simulink model "filling_model"  (R2020b)
settings: Solver=FixedStepAuto  StartTime=tank_pressure.time(1)  StopTime=tank_pressure.time(end)  FixedStep=1  RelTol=1e-3
undefined symbols (not defined in the file or in its folder): bar_to_Pa, eta_Faraday_builtin, F, k, ncell, R, tank_pressure, Ttank, Vtank
settings Model: Creator=keske  LastModifiedBy=keske

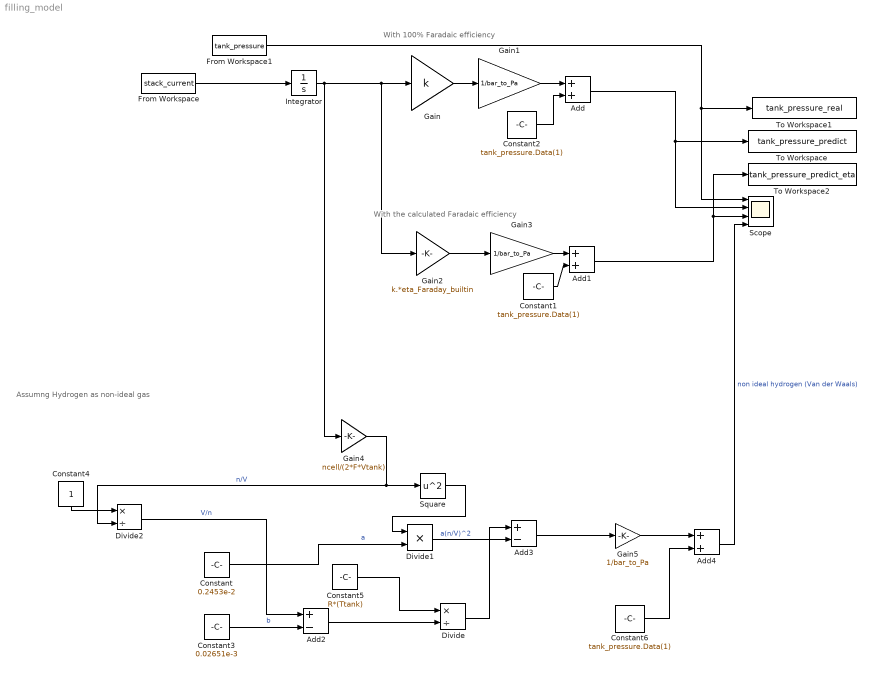
== system filling_model ==
  note: With 100% Faradaic efficiency
  note: With the calculated Faradaic efficiency
  note: Assumng Hydrogen as non-ideal gas
  Add : Sum
  Add1 : Sum
  Add2 : Sum  Inputs=+-
  Add3 : Sum  Inputs=+-
  Add4 : Sum
  Constant : Constant  Value=0.2453e-2
  Constant1 : Constant  Value=tank_pressure.Data(1)
  Constant2 : Constant  Value=tank_pressure.Data(1)
  Constant3 : Constant  Value=0.02651e-3
  Constant4 : Constant
  Constant5 : Constant  Value=R*(Ttank)  VectorParams1D=off
  Constant6 : Constant  Value=tank_pressure.Data(1)
  Divide : Product  Inputs=*/
  Divide1 : Product  Inputs=**
  Divide2 : Product  Inputs=*/
  From Workspace : FromWorkspace  VariableName=stack_current  SampleTime=1  OutputAfterFinalValue=Holding final value
  From Workspace1 : FromWorkspace  VariableName=tank_pressure  SampleTime=1
  Gain : Gain  Gain=k
  Gain1 : Gain  Gain=1/bar_to_Pa
  Gain2 : Gain  Gain=k.*eta_Faraday_builtin
  Gain3 : Gain  Gain=1/bar_to_Pa
  Gain4 : Gain  Gain=ncell/(2*F*Vtank)
  Gain5 : Gain  Gain=1/bar_to_Pa
  Integrator : Integrator
  Scope : Scope  NumInputPorts=4
  Square : Math  Operator=square  SaturateOnIntegerOverflow=on
  To Workspace : ToWorkspace  VariableName=tank_pressure_predict  SaveFormat=Timeseries  SampleTime=-1
  To Workspace1 : ToWorkspace  VariableName=tank_pressure_real  SaveFormat=Timeseries  SampleTime=-1
  To Workspace2 : ToWorkspace  VariableName=tank_pressure_predict_eta  SaveFormat=Timeseries  SampleTime=-1
  wires:
  Constant2/1 -> Add/2
  Gain/1 -> Gain1/1
  From Workspace1/1 -> To Workspace1/1, Scope/1
  From Workspace/1 -> Integrator/1
  Gain1/1 -> Add/1
  Constant1/1 -> Add1/2
  Gain3/1 -> Add1/1
  Gain2/1 -> Gain3/1
  Integrator/1 -> Gain4/1, Gain2/1, Gain/1
  Add1/1 -> To Workspace2/1, Scope/3
  Add/1 -> Scope/2, To Workspace/1
  Constant/1 -> Divide1/2  "a"
  Constant3/1 -> Add2/2  "b"
  Gain4/1 -> Divide2/2, Square/1  "n/V"
  Square/1 -> Divide1/1
  Divide1/1 -> Add3/2  "a(n/V)^2"
  Constant4/1 -> Divide2/1
  Divide2/1 -> Add2/1  "V/n"
  Constant5/1 -> Divide/1
  Add2/1 -> Divide/2
  Divide/1 -> Add3/1
  Add3/1 -> Gain5/1
  Gain5/1 -> Add4/1
  Constant6/1 -> Add4/2
  Add4/1 -> Scope/4  "non ideal hydrogen (Van der Waals)"
